simulink model "Copy_2_of_calibration_sensors"  (R2026a)
settings: Solver=FixedStepDiscrete  StopTime=inf  FixedStep=0.01
StopFcn:
  | coefficients = out.coefficients;
  | 
  | folder = 'calibration_data';
  | 
  | if ~exist(folder, 'dir')
  |     mkdir(folder);
  | end
  | 
  | baseName = 'sensor_calibration';
  | fileName = fullfile(folder, baseName + ".mat");
  | 
  | n = 2;
  | 
  | while exist(fileName, 'file')
  |     fileName = fullfile(folder, ...
  |         baseName + "_" + n + ".mat");
  |     n = n + 1;
  | end
  | 
  | save(fileName, 'coefficients');
  | 
  | fprintf('Calibration saved to: %s\n', fileName);
(part 4 of 4)

== matlab function Copy_2_of_calibration_sensors/MATLAB Function ==
  data: finished1 output; finished2 output; finished3 output; coef output; conflevel1 input; conflevel2 input; conflevel3 input; conflevel4 input; conflevel5 input; conflevel6 input; conflevel7 input; conflevel8 input; conflevel9 input; adc1 input; adc2 input; adc3 input
function [finished1, finished2, finished3, coef] = fcn( ...
    conflevel1, conflevel2, conflevel3, ...
    conflevel4, conflevel5, conflevel6, ...
    conflevel7, conflevel8, conflevel9, ...
    adc1, adc2, adc3)

persistent adc_pts h_pts done last_btn

N = 9;

if isempty(adc_pts)
    adc_pts = zeros(3, N);
    h_pts   = zeros(3, N);

    done = zeros(1, N);

    last_btn = zeros(N, 1);
end

btn = [ ...
    conflevel1;
    conflevel2;
    conflevel3;
    conflevel4;
    conflevel5;
    conflevel6;
    conflevel7;
    conflevel8;
    conflevel9
    ];

edge = (btn == 1) & (last_btn == 0);
last_btn = btn;

levels = [10 15 20 25 30 35 40 45 50];

for k = 1:N

    if edge(k)

        adc_pts(1,k) = adc1;
        adc_pts(2,k) = adc3;
        adc_pts(3,k) = adc2;

        h_pts(:,k) = levels(k);

        done(k) = 1;

    end

end

coef = zeros(3,4);

if sum(done) == N

    for i = 1:3

        x = adc_pts(i,:)';
        y = h_pts(i,:)';

        X = [x.^3, x.^2, x, ones(N,1)];

        p = X \ y;

        coef(i,:) = p';

    end

end

finished = sum(done) == N;

finished1 = finished;
finished2 = finished;
finished3 = finished;

end
